simulink model "DC_MotorSim"  (Simulink 8.7)
settings: Solver=ode5  StartTime=0.0  StopTime=2  FixedStep=0.0001  RelTol=1e-3
undefined symbols (not defined in the file): C, J, Kb, Kt, L, R, Tf
libraries: simulink x1
settings Model: Creator=010796305  LastModifiedBy=010796305
settings DataIOCC: LimitDataPoints=off  SaveFormat=Dataset
settings DebuggingCC: UnderspecifiedInitializationDetection=Simplified  MergeDetectMultiDrivingBlocksExec=error
settings HardwareCC: ProdBitPerPointer=64  ProdLargestAtomicFloat=Float  ProdIntDivRoundTo=Zero  ProdEndianess=LittleEndian  ProdWordSize=64  ProdHWDeviceType=Intel->x86-64 (Windows64)
settings ModelReferenceCC: PropagateSignalLabelsOutOfModel=on
settings ConfigComp: CovModelRefEnable=off

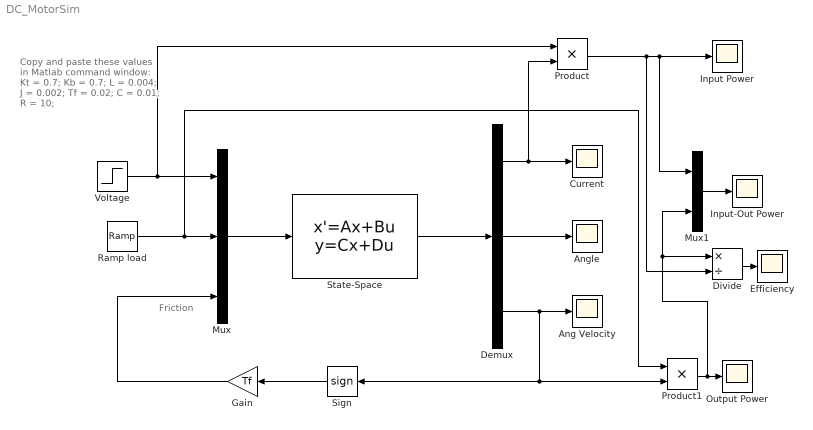
== system DC_MotorSim ==
  note: Copy and paste these values  in Matlab command window:
      |
      | Kt = 0.7;
      | Kb = 0.7;
      | L = 0.004;
      | J = 0.002;
      | Tf = 0.02;
      | C = 0.01;
      | R = 10;
  note: Friction
  Ang Velocity : Scope
  Angle : Scope
  Current : Scope
  Demux : Demux  Outputs=3
  Divide : Product  Inputs=*/
  Efficiency : Scope
  Gain : Gain  Gain=Tf
  Input Power : Scope
  Input-Out Power : Scope
  Mux : Mux  Inputs=3
  Mux1 : Mux  Inputs=2
  Output Power : Scope
  Product : Product
  Product1 : Product
  Ramp load : simulink/Sources/Ramp  slope=0.05  start=1  X0=0
  Sign : Signum
  State-Space : StateSpace  A=[-R/L 0 -Kb/L; 0 0 1; Kt/J 0 -C/J]  B=[1/L 0 0; 0 0 0; 0 -1/J -1/J]  C=eye(3)  D=zeros(3,3)  X0=0
  Voltage : Step  Time=0  SampleTime=0
  wires:
  Mux/1 -> State-Space/1
  State-Space/1 -> Demux/1
  Demux/1 -> Product/2, Current/1
  Demux/2 -> Angle/1
  Demux/3 -> Product1/2, Sign/1, Ang Velocity/1
  Product/1 -> Divide/2, Mux1/1, Input Power/1
  Sign/1 -> Gain/1
  Gain/1 -> Mux/3
  Voltage/1 -> Product/1, Mux/1
  Ramp load/1 -> Mux/2, Product1/1
  Mux1/1 -> Input-Out Power/1
  Product1/1 -> Divide/1, Mux1/2, Output Power/1
  Divide/1 -> Efficiency/1
